simulink model "PID_inverseDynamics"  (R2016a)
settings: Solver=VariableStepAuto  StartTime=0.0  StopTime=4  FixedStep=0.01  RelTol=1e-3
libraries: simulink x4
settings Model: Creator=FPCC  LastModifiedBy=FPCC

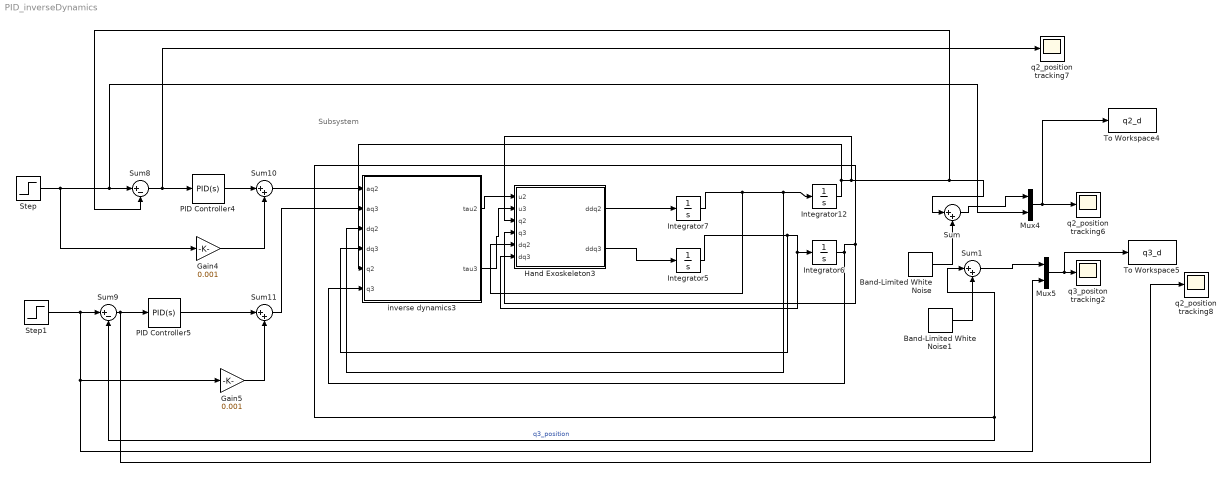
== system PID_inverseDynamics ==
  note: Subsystem
  Band-Limited White Noise : simulink/Sources/Band-Limited White Noise  Cov=[0.01]  Ts=0.1  seed=[23341]
  Band-Limited White Noise1 : simulink/Sources/Band-Limited White Noise  Cov=[0.01]  Ts=0.1  seed=[23341]
  Gain4 : Gain  Gain=0.001
  Gain5 : Gain  Gain=0.001
  Hand Exoskeleton3 : MATLAB Function  TreatAsAtomicUnit=on
  Integrator{5..7,12} (4 alike) : Integrator
  Mux4 : Mux  Inputs=2
  Mux5 : Mux  Inputs=2
  PID Controller4 : simulink/Continuous/PID Controller  Controller=PID  TimeDomain=Continuous-time  SampleTime=-1  IntegratorMethod=Forward Euler  FilterMethod=Forward Euler  Form=Parallel  UseFilter=on  ControllerParametersSource=internal  P=262.466504109675  I=153.121092161281  D=99.9617214848896  N=11428.279760416  InitialConditionSource=internal  InitialConditionForIntegrator=0  InitialConditionForFilter=0  ExternalReset=none  LimitOutput=off  UpperSaturationLimit=inf  LowerSaturationLimit=-inf  LinearizeAsGain=on  AntiWindupMode=none  Kb=1  TrackingMode=off  Kt=1  PParamMin=[]  PParamMax=[]  IParamMin=[]  IParamMax=[]  DParamMin=[]  DParamMax=[]  NParamMin=[]  NParamMax=[]  KbParamMin=[]  KbParamMax=[]  KtParamMin=[]  KtParamMax=[]  POutMin=[]  POutMax=[]  IOutMin=[]  IOutMax=[]  DOutMin=[]  DOutMax=[]  NOutMin=[]  NOutMax=[]  KbOutMin=[]  KbOutMax=[]  KtOutMin=[]  KtOutMax=[]  IntegratorOutMin=[]  IntegratorOutMax=[]  FilterOutMin=[]  FilterOutMax=[]  SumOutMin=[]  SumOutMax=[]  SumI1OutMin=[]  SumI1OutMax=[]  SumI2OutMin=[]  SumI2OutMax=[]  SumI3OutMin=[]  SumI3OutMax=[]  SumDOutMin=[]  SumDOutMax=[]  SaturationOutMin=[]  SaturationOutMax=[]  IntegratorContinuousStateAttributes=''  IntegratorStateMustResolveToSignalObject=off  IntegratorRTWStateStorageClass=Auto  FilterContinuousStateAttributes=''  FilterStateMustResolveToSignalObject=off  FilterRTWStateStorageClass=Auto  DifferentiatorICPrevScaledInput=0  DifferentiatorOutMin=[]  DifferentiatorOutMax=[]
  PID Controller5 : simulink/Continuous/PID Controller  Controller=PID  TimeDomain=Continuous-time  SampleTime=-1  IntegratorMethod=Forward Euler  FilterMethod=Forward Euler  Form=Parallel  UseFilter=on  ControllerParametersSource=internal  P=262.466504114729  I=153.12109216423  D=99.9617214868145  N=11428.279760416  InitialConditionSource=internal  InitialConditionForIntegrator=0  InitialConditionForFilter=0  ExternalReset=none  LimitOutput=off  UpperSaturationLimit=inf  LowerSaturationLimit=-inf  LinearizeAsGain=on  AntiWindupMode=none  Kb=1  TrackingMode=off  Kt=1  PParamMin=[]  PParamMax=[]  IParamMin=[]  IParamMax=[]  DParamMin=[]  DParamMax=[]  NParamMin=[]  NParamMax=[]  KbParamMin=[]  KbParamMax=[]  KtParamMin=[]  KtParamMax=[]  POutMin=[]  POutMax=[]  IOutMin=[]  IOutMax=[]  DOutMin=[]  DOutMax=[]  NOutMin=[]  NOutMax=[]  KbOutMin=[]  KbOutMax=[]  KtOutMin=[]  KtOutMax=[]  IntegratorOutMin=[]  IntegratorOutMax=[]  FilterOutMin=[]  FilterOutMax=[]  SumOutMin=[]  SumOutMax=[]  SumI1OutMin=[]  SumI1OutMax=[]  SumI2OutMin=[]  SumI2OutMax=[]  SumI3OutMin=[]  SumI3OutMax=[]  SumDOutMin=[]  SumDOutMax=[]  SaturationOutMin=[]  SaturationOutMax=[]  IntegratorContinuousStateAttributes=''  IntegratorStateMustResolveToSignalObject=off  IntegratorRTWStateStorageClass=Auto  FilterContinuousStateAttributes=''  FilterStateMustResolveToSignalObject=off  FilterRTWStateStorageClass=Auto  DifferentiatorICPrevScaledInput=0  DifferentiatorOutMin=[]  DifferentiatorOutMax=[]
  Step : Step  Time=0  SampleTime=0
  Step1 : Step  Time=0  SampleTime=0
  Sum{,1,10..11} (4 alike) : Sum  Inputs=|++
  Sum8 : Sum  Inputs=|+-
  Sum9 : Sum  Inputs=|+-
  To Workspace4 : ToWorkspace  VariableName=q2_d  SaveFormat=Timeseries  SampleTime=-1
  To Workspace5 : ToWorkspace  VariableName=q3_d  SaveFormat=Timeseries  SampleTime=-1
  inverse dynamics3 : MATLAB Function  TreatAsAtomicUnit=on
  q2_position tracking6 : Scope
  q2_position tracking7 : Scope
  q2_position tracking8 : Scope
  q3_positon tracking2 : Scope
  wires:
  Step/1 -> Gain4/1, Sum8/1, Mux4/2
  Sum9/1 -> PID Controller5/1, q2_position tracking8/1
  Integrator12/1 -> Hand Exoskeleton3/3(q2), Sum/1, Sum8/2, inverse dynamics3/5(q2)
  Integrator6/1 -> inverse dynamics3/6(q3), Hand Exoskeleton3/4(q3), Sum1/1, Sum9/2  "q3_position"
  PID Controller4/1 -> Sum10/1
  Step1/1 -> Sum9/1, Gain5/1, Mux5/2
  Mux5/1 -> To Workspace5/1, q3_positon tracking2/1
  Mux4/1 -> To Workspace4/1, q2_position tracking6/1
  Gain4/1 -> Sum10/2
  Gain5/1 -> Sum11/2
  Sum11/1 -> inverse dynamics3/2(aq3)
  Hand Exoskeleton3/1(ddq2) -> Integrator7/1
  inverse dynamics3/2(tau3) -> Hand Exoskeleton3/2(u3)
  Integrator7/1 -> Integrator12/1, inverse dynamics3/3(dq2), Hand Exoskeleton3/5(dq2)
  Hand Exoskeleton3/2(ddq3) -> Integrator5/1
  Integrator5/1 -> Hand Exoskeleton3/6(dq3), Integrator6/1, inverse dynamics3/4(dq3)
  inverse dynamics3/1(tau2) -> Hand Exoskeleton3/1(u2)
  Sum10/1 -> inverse dynamics3/1(aq2)
  Sum8/1 -> q2_position tracking7/1, PID Controller4/1
  PID Controller5/1 -> Sum11/1
  Band-Limited White Noise/1 -> Sum/2
  Sum/1 -> Mux4/1
  Band-Limited White Noise1/1 -> Sum1/2
  Sum1/1 -> Mux5/1

== matlab function PID_inverseDynamics/Hand Exoskeleton3 ==
  data: u2 input; u3 input; q2 input; ddq2 output; q3 input; ddq3 output; dq2 input; dq3 input
function [ddq2,ddq3] = fcn(u2,u3,q2,q3,dq2,dq3)
L1 = 12; L2 = 20; L3 = 45; L4 = 15; L5 = 20;
m1 = 100; m2 = 70; m3 = 170; m4 = 100; m5 = 20;
I1 = 1; I2 = 1; I3 = 1; I4 = 1; I5 = 1;

V=47;
H=20;

q1 = (L1 - V) * tan(q2);




% A = V - L1 - (L2 + L3*cos(q3)) * cos(q2);
% B = (H - L3*sin(q3)) * cos(q2);
% C = L4 * cos(q2);
% R = sqrt(A^2 + B^2-C^2);
% phi = atan2(A, B);
% 
% 
% dA=L2*sin(q2)*dq2-L3*(sin(q3)*cos(q2)*dq3+cos(q3)*sin(q2)*dq2);
% dB=L3*(sin(q3)*sin(q2)*dq2-cos(q3)*cos(q2)*dq3)-H*sin(q2)*dq2;
% dC=-L4*sin(q2)*dq2;
% 
% dR=(A*dA+dB*B-C*dC)/R;
% dphi=(dA*B-dB*A)/(B^2)/(1+(A/B)^2);
% 
% 
% 
% qtemp1 = atan2(C , R) - phi;
% %qtemp2 = -acos(C / R) + phi;
% q4 = qtemp1 - q3;
% dq4=(C*dR-dC*R)/(R^2)/(1+(C/R)^2)+ dphi - dq3;
q4=q3;
dq4=dq3;

q5=(H-L4*cos(q3+q4)-L3*cos(q3))/cos(q3+q4);
dq5=(L3*sin(q3)*dq3*cos(q3+q4)+sin(q3+q4)*(dq3+dq4)*(H-L3*cos(q3)))/cos(q3+q4)^2;




% Inertia matrices (placeholders, replace with actual inertia tensors)
%

% Gravitational acceleration
g = 9.82;

M=[m2*L1^2-I2*cos(q2) 0;
    0 L2^2*m3-I3*cos(q3)+I3*cos(q2)^2+I3*cos(q2)^2*cos(q3)];
invM=inv(M);
C=[ (I2*dq2^2*sin(q2))/2 + (I3*dq3^2*sin(2*q2))/2 - (I5*dq5^2*sin(2*q2))/2 - (I4*dq4^2*cos(q2)*sin(q4))/2 - (I4*dq4^2*cos(q4)*sin(q2))/2 + (I4*dq4^2*cos(q2)*cos(q3)^2*sin(q4))/2 + (I4*dq4^2*cos(q3)^2*cos(q4)*sin(q2))/2 + I5*dq5^2*cos(q2)*cos(q3)^2*sin(q2) - (I5*dq5^2*cos(q2)*cos(q3)^2*sin(q4))/2 + I3*dq3^2*cos(q2)*cos(q3)*sin(q2) - (I5*dq5^2*cos(q3)*cos(q4)*sin(q2))/2 - (I5*dq5^2*cos(q3)*cos(q4)*sin(q3))/2 + I5*dq5^2*cos(q2)^2*cos(q3)*cos(q4)*sin(q3) - I5*dq5^2*cos(q2)*sin(q2)*sin(q3)*sin(q4);
 (I3*dq3^2*sin(q3))/2 + (I4*dq4^2*sin(2*q3))/2 - (I5*dq5^2*sin(2*q3))/2 - (I3*dq3^2*cos(q2)^2*sin(q3))/2 - I3*dq2*dq3*sin(2*q2) + I5*dq5^2*cos(q2)^2*cos(q3)*sin(q3) + (I5*dq5^2*cos(q2)^2*cos(q3)*sin(q4))/2 - (I5*dq5^2*cos(q2)*cos(q4)*sin(q2))/2 - (I5*dq5^2*cos(q2)*cos(q4)*sin(q3))/2 + I5*dq5^2*cos(q2)*cos(q3)^2*cos(q4)*sin(q2) + I4*dq4^2*cos(q2)*cos(q3)*cos(q4)*sin(q3) - I4*dq4^2*cos(q3)*sin(q2)*sin(q3)*sin(q4) + I5*dq5^2*cos(q3)*sin(q2)*sin(q3)*sin(q4) - 2*I3*dq2*dq3*cos(q2)*cos(q3)*sin(q2)];

G=[0;
 g*cos(q3)*(L2*m3 + L2*m4 + L2*m5 + L3*m4*cos(q4) + L3*m5*cos(q4) + L4*m5*cos(q4))];
ddq=[0;0];
ddq=invM*([u2;u3]-C-G);
ddq2=ddq(1);
ddq3=ddq(2);

== matlab function PID_inverseDynamics/inverse dynamics3 ==
  data: aq2 input; tau2 output; aq3 input; dq2 input; dq3 input; tau3 output; q2 input; q3 input
function [tau2,tau3] = fcn(aq2,aq3,dq2,dq3,q2,q3)


L1 = 12; L2 = 20; L3 = 45; L4 = 15; L5 = 20;
m1 = 100; m2 = 70; m3 = 170; m4 = 100; m5 = 20;
I1 = 1; I2 = 1; I3 = 1; I4 = 1; I5 = 1;

V=47;
H=20;
ddq2=aq2;
ddq3=aq3;

q1 = (L1 - V) * tan(q2);



% A = V - L1 - (L2 + L3*cos(q3)) * cos(q2);
% B = (H - L3*sin(q3)) * cos(q2);
% C = L4 * cos(q2);
% R = sqrt(A^2 + B^2-C^2);
% phi = atan2(A, B);
% 
% 
% dA=L2*sin(q2)*dq2-L3*(sin(q3)*cos(q2)*dq3+cos(q3)*sin(q2)*dq2);
% dB=L3*(sin(q3)*sin(q2)*dq2-cos(q3)*cos(q2)*dq3)-H*sin(q2)*dq2;
% dC=-L4*sin(q2)*dq2;
% 
% dR=(A*dA+dB*B-C*dC)/R;
% dphi=(dA*B-dB*A)/(B^2)/(1+(A/B)^2);
% 
% 
% 
% qtemp1 = atan2(C , R) - phi;
% %qtemp2 = -acos(C / R) + phi;
% q4 = qtemp1 - q3;
% dq4=(C*dR-dC*R)/(R^2)/(1+(C/R)^2)+ dphi - dq3;
q4=q3;
dq4=dq3;
q5=(H-L4*cos(q3+q4)-L3*cos(q3))/cos(q3+q4);
dq5=(L3*sin(q3)*dq3*cos(q3+q4)+sin(q3+q4)*(dq3+dq4)*(H-L3*cos(q3)))/cos(q3+q4)^2;



ddq = [ ddq2; ddq3;];


% Inertia matrices (placeholders, replace with actual inertia tensors)
%

% Gravitational acceleration
g = 9.82;
M=[m2*L1^2-I2*cos(q2) 0;
    0 L2^2*m3-I3*cos(q3)+I3*cos(q2)^2+I3*cos(q2)^2*cos(q3)];
invM=inv(M);
C=[ (I2*dq2^2*sin(q2))/2 + (I3*dq3^2*sin(2*q2))/2 - (I5*dq5^2*sin(2*q2))/2 - (I4*dq4^2*cos(q2)*sin(q4))/2 - (I4*dq4^2*cos(q4)*sin(q2))/2 + (I4*dq4^2*cos(q2)*cos(q3)^2*sin(q4))/2 + (I4*dq4^2*cos(q3)^2*cos(q4)*sin(q2))/2 + I5*dq5^2*cos(q2)*cos(q3)^2*sin(q2) - (I5*dq5^2*cos(q2)*cos(q3)^2*sin(q4))/2 + I3*dq3^2*cos(q2)*cos(q3)*sin(q2) - (I5*dq5^2*cos(q3)*cos(q4)*sin(q2))/2 - (I5*dq5^2*cos(q3)*cos(q4)*sin(q3))/2 + I5*dq5^2*cos(q2)^2*cos(q3)*cos(q4)*sin(q3) - I5*dq5^2*cos(q2)*sin(q2)*sin(q3)*sin(q4);
 (I3*dq3^2*sin(q3))/2 + (I4*dq4^2*sin(2*q3))/2 - (I5*dq5^2*sin(2*q3))/2 - (I3*dq3^2*cos(q2)^2*sin(q3))/2 - I3*dq2*dq3*sin(2*q2) + I5*dq5^2*cos(q2)^2*cos(q3)*sin(q3) + (I5*dq5^2*cos(q2)^2*cos(q3)*sin(q4))/2 - (I5*dq5^2*cos(q2)*cos(q4)*sin(q2))/2 - (I5*dq5^2*cos(q2)*cos(q4)*sin(q3))/2 + I5*dq5^2*cos(q2)*cos(q3)^2*cos(q4)*sin(q2) + I4*dq4^2*cos(q2)*cos(q3)*cos(q4)*sin(q3) - I4*dq4^2*cos(q3)*sin(q2)*sin(q3)*sin(q4) + I5*dq5^2*cos(q3)*sin(q2)*sin(q3)*sin(q4) - 2*I3*dq2*dq3*cos(q2)*cos(q3)*sin(q2)];

G=[0;
 g*cos(q3)*(L2*m3 + L2*m4 + L2*m5 + L3*m4*cos(q4) + L3*m5*cos(q4) + L4*m5*cos(q4))];

tau = M * ddq + C + G;
tau2=tau(1);
tau3=tau(2);
